simulink model "wifi_1"  (R2023b)
settings: Solver=VariableStepDiscrete  StartTime=0.0  StopTime=1000  RelTol=1e-3
values from neighbouring files (symbols this model uses):
  shift = (2*pi*radial_v*symbol_duration)/lambda_subc    [base_5G_test_env_base.m]    (also in wifi_doppler.m = zeros(1,length(f_x)))
libraries: simulink x2, commdigbbndam3 x2, commchan3 x1, commutil2 x1, commsink2 x1, commrflib2 x1, commrandsrc3 x1
settings Model: Creator=loisb  LastModifiedBy=loisb
settings SolverCC: AlgebraicLoopSolver=TrustRegion  AutoInsertRateTranBlk=on
settings DataIOCC: ExternalInput=sim_phase_shift.getElement(1)  LimitDataPoints=on  SaveTime=off
settings OptimizationCC: BooleanDataType=off  DefaultParameterBehavior=Inlined  LocalBlockOutputs=off  LifeSpan=inf
settings DebuggingCC: AlgebraicLoopMsg=error  SingleTaskRateTransMsg=error  UnconnectedInputMsg=warning  UnconnectedOutputMsg=warning  UnconnectedLineMsg=warning  AllowSymbolicDim=off  SFUnexpectedBacktrackingDiag=warning  SFNoUnconditionalDefaultTransitionDiag=warning  SFExecutionAtInitializationDiag=none  ArithmeticOperatorsInVariantConditions=warning
settings ModelReferenceCC: EnableRefExpFcnMdlSchedulingChecks=on
settings SFSimCC: SimUseLocalCustomCode=off  CustomCodeUndefinedFunction=UseInterfaceOnly
settings RTWCC: RTWUseLocalCustomCode=off
settings CodeAppCC: StateflowObjectComments=on
settings GRTTargetCC: TargetLangStandard=C89/C90 (ANSI)
settings ConfigComp: CovMetricSettings=dw  CovSaveCumulativeToWorkspaceVar=on  CovSaveSingleToWorkspaceVar=on  CovExternalEMLEnable=off  CovSFcnEnable=off

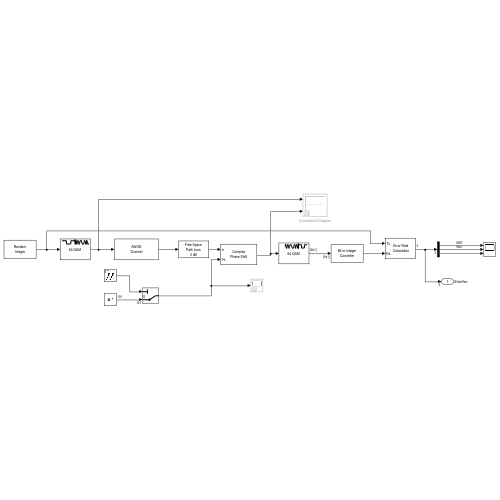
[thumbnail: Simulink's stored preview of the top-level diagram]
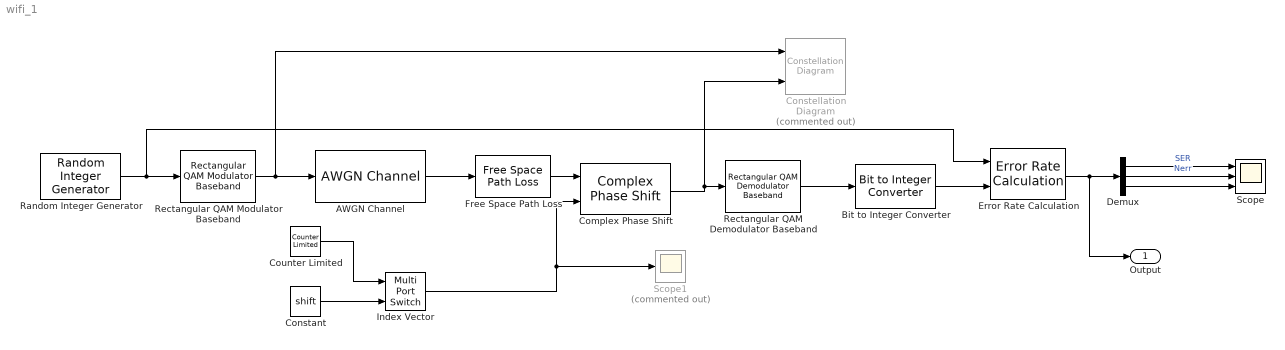
== system wifi_1 ==
  AWGN Channel : commchan3/AWGN Channel  LegacyMode=off  NoiseMethod="Signal to noise ratio  (SNR)"  noiseMode="Signal to noise ratio  (SNR)"  EbNo=10  EsNo=10  SNR=15  BitsPerSymbol=1  SignalPower=1  SamplesPerSymbol=1  SymbolPeriod=1  VarianceSource=Parameter  Variance=1  RandomStream=Global stream  Seed=67  SimulateUsing=Code generation
  Bit to Integer Converter : simulink/Logic and Bit Operations/Bit to Integer Converter  nbits=6  bitOrder=MSB first  signedOutputValues=Unsigned  outDtype=Inherit via internal rule  outDtypeSigned=Inherit via internal rule
      settings: LibrarySourceBlock=|
      | commutil2/Bit to Integer
      | Converter
  Complex Phase Shift : commutil2/Complex Phase Shift
  Constant : Constant  Value=shift
  Constellation Diagram : ConstellationDiagram  Commented=on  NumInputPorts=2  WindowPosition=[1.000000,49.000000,1536.000000,793.000000,]  Visible=on  ScopeFrameLocation=window  SymbolsToDisplaySource=Property  SymbolsToDisplay=1000  ReferenceConstellation="{[-7+7i  -7+5i  -7+3i  -7+1i  -7-1i  -7-3i  -7-5i  -7-7i  -5+7i  -5+5i  -5+3i  -5+1i  -5-1i  -5-3i  -5-5i  -5-7i  -3+7i  -3+5i  -3+3i  -3+1i  -3-1i  -3-3i  -3-5i  -3-7i  -1+7i  -1+5i  -1+3i  -1+1i  -1-1i  -1-3i  -1-5i  -1-7i   1+7i   1+5i   1+3i   1+1i   1-1i   1-3i   1-5i   1-7i   3+7i   3+5i   3+3i   3+1i   3-1i   3-3i   3-5i   3-7i   5+7i   5+5i   5+3i   5+1i   5-1i   5-3i   5-5i   5-7i   7+7i   7+5i   7+3i   7+1i   7-1i   7-3i   7-5i   7-7i][0.7071+0.7071i          -0.7071+0.7071i          -0.7071-0.7071i            0.707-0.7071i]}"  XLimits=[-211.84,224.28]  YLimits=[-104.73,102.61]  ShowLegend=on  ShowReferenceConstellation=off  EnableMeasurements=on
  Counter Limited : simulink/Sources/Counter Limited  uplimit=101  tsamp=10
  Demux : Demux  Outputs=3
  Error Rate Calculation : commsink2/Error Rate Calculation  N=0  st_delay=0  cp_mode=Entire frame  subframe=[]  PMode=Port  WsName=ErrorVec  RsMode2=off  stop=off  numErr=100  maxBits=1e6
  Free Space Path Loss : commrflib2/Free Space Path Loss  mode=Decibels  dB=3  d=0.005  fc=2.4e9
  Index Vector : MultiPortSwitch  DataPortOrder=Zero-based contiguous  Inputs=1  zeroidx=on  SaturateOnIntegerOverflow=off  InputSameDT=off
  Random Integer Generator : commrandsrc3/Random Integer Generator  SetSize=64  SeedSource=Auto  Seed=0  SampleTime=1  SamplesPerFrame=1  OutputDataType=double  SimulateUsing=Interpreted execution
  Rectangular QAM Demodulator Baseband : commdigbbndam3/Rectangular QAM Demodulator Baseband  M=64  OutType=Bit  DecType=Hard decision  VarSource=Dialog  Variance=1  Dec=Gray  Mapping=[0:15]  PowType=Min. distance between symbols  MinDist=2  AvgPow=1  PeakPow=1  Ph=0  outDtype1=Inherit via internal rule  outDtype2=Inherit via internal rule  derotateFactorWordLen=16  derotateFactorDataTypeStr=Inherit: Same word length as input  derotateFactorLastDataTypeStr=Inherit: Same word length as input  denormFactorWordLen=16  denormFactorDataTypeStr=Inherit: Same word length as input  denormFactorLastDataTypeStr=Inherit: Same word length as input  prodOutWordLen=32  prodOutOverflowMode=Wrap  prodOutRoundingMode=Floor  prodOutOvFlMode=off  prodOutOvFlModeLastStrValue=off  sumWordLen=32
  Rectangular QAM Modulator Baseband : commdigbbndam3/Rectangular QAM Modulator Baseband  M=64  InType=Integer  Enc=Gray  Mapping=[0:15]  PowType=Min. distance between symbols  MinDist=2  AvgPow=1  PeakPow=1  Ph=0  outDtype=double  outWordLen=16  outUDDataType=sfix(16)  outFracLenMode=Best precision  outFracLen=15  outDataTypeStr=double  outLastDataTypeStr=double
  Scope : Scope  NumInputPorts=3
  Scope1 : Scope  Commented=on
  Output : Outport  SignalName=ErrorVec
  wires:
  Rectangular QAM Modulator Baseband/1 -> Constellation Diagram/1, AWGN Channel/1
  AWGN Channel/1 -> Free Space Path Loss/1
  Complex Phase Shift/1 -> Constellation Diagram/2, Rectangular QAM Demodulator Baseband/1
  Random Integer Generator/1 -> Error Rate Calculation/1, Rectangular QAM Modulator Baseband/1
  Error Rate Calculation/1 -> Output/1, Demux/1
  Demux/1 -> Scope/1  "SER"
  Demux/2 -> Scope/2  "Nerr"
  Demux/3 -> Scope/3
  Bit to Integer Converter/1 -> Error Rate Calculation/2
  Rectangular QAM Demodulator Baseband/1 -> Bit to Integer Converter/1
  Free Space Path Loss/1 -> Complex Phase Shift/1
  Constant/1 -> Index Vector/2
  Index Vector/1 -> Scope1/1, Complex Phase Shift/2
  Counter Limited/1 -> Index Vector/1
